simulink model "UdpHost"  (R2016b)
settings: Solver=FixedStepDiscrete  StartTime=0.0  StopTime=inf  FixedStep=CassieParameters.etherCatSampleTime  RelTol=1e-3  EnableMultiTasking=on
InitFcn:
  | udpInitFcn;
undefined symbols (not defined in the file or in its folder): inputBytes, outputBytes
libraries: ptplib x3, xpcutilitieslib x2
settings Model: xpc_rtwmakecfg_data=_xpciplib__xpcnblib__xpcetherlib__xpcether8255xlib__xpcetherGbElib_  SimulationMode=external  Creator=robot  LastModifiedBy=mikha
settings SolverCC: EnableConcurrentExecution=on  ConcurrentTasks=on
settings DataIOCC: SaveFormat=Array  SaveOutput=off  SignalLogging=off  DSMLogging=off  VisualizeSimOutput=off  SaveTime=off
settings OptimizationCC: DefaultParameterBehavior=Inlined  OptimizeBlockIOStorage=off  BufferReuse=off  GlobalBufferReuse=off  ExpressionFolding=off  LocalBlockOutputs=off  LifeSpan=inf  SimCompilerOptimization=on  AccelVerboseBuild=on
settings DebuggingCC: AllowSymbolicDim=off  SFUnexpectedBacktrackingDiag=warning  SFNoUnconditionalDefaultTransitionDiag=warning  SFExecutionAtInitializationDiag=none
settings HardwareCC: ProdBitPerPointer=32  ProdBitPerSizeT=32  ProdBitPerPtrDiffT=32  ProdLargestAtomicFloat=None  ProdWordSize=32  ProdLongLongMode=on  ProdHWDeviceType=Generic->32-bit x86 compatible
settings ModelReferenceCC: EnableParallelModelReferenceBuilds=on  ParallelModelReferenceMATLABWorkerInit=Copy Base Workspace  ModelReferenceNumInstancesAllowed=Zero  PropagateSignalLabelsOutOfModel=off
settings SFSimCC: SFSimEcho=off
settings RTWCC: SystemTargetFile=slrt.tlc  TLCOptions=-axPCMaxOverloads=1000000000 -axPCMaxOverloadLen=1000000000  TemplateMakefile=slrt_default_tmf  Description=Simulink Real-Time  RTWCompilerOptimization=on
settings CodeAppCC: GenerateComments=off  SimulinkBlockComments=off
settings SimulinkRealTimeCC: xPCTargetPCEnvName=NUC
settings ConfigComp: CovMetricSettings=dw  CovHtmlReporting=on  CovSaveCumulativeToWorkspaceVar=on  CovSaveSingleToWorkspaceVar=on  CovExternalEMLEnable=off

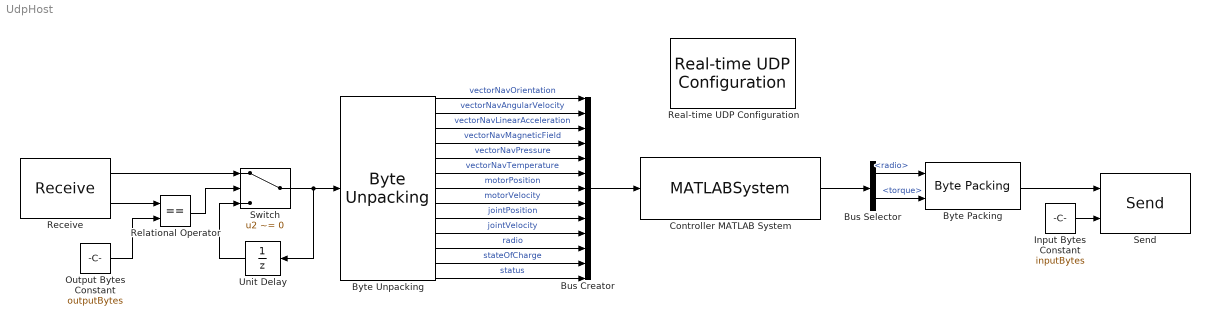
== system UdpHost ==
  Bus Creator : BusCreator  Inputs=13  OutDataTypeStr=Bus: cassieOutputsBus
  Bus Selector : BusSelector  OutputSignals=radio,torque
  "Byte Packing " : xpcutilitieslib/Byte Packing   MaskPackedDataType=uint8  MaskUnpackedDataTypes=inputTypes  MaskAlignment=1
  "Byte Unpacking " : xpcutilitieslib/Byte Unpacking   MaskUnpackedDataTypes=outputTypes  MaskUnpackedDataSizes=outputSizes  MaskAlignment=1
  Controller MATLAB System : MATLABSystem  System=NullController  SimulateUsing=Code generation
      mask Type: NullController
      mask Display:
      | disp('NullController');
      | port_label('input',1,'outputs');
      | port_label('output',1,'inputs');
  Input Bytes Constant : Constant  Value=inputBytes
  Output Bytes Constant : Constant  Value=outputBytes
  "Real-time UDP Configuration " : ptplib/PTP UDP/Real-time UDP  Configuration   ID=1  IpAddress=10.10.10.2  SubnetMask=255.255.255.0  Gateway=0.0.0.0  EthDrv=Intel Gigabit  PciBus=3  PciSlot=0  udpID=0  MulticastList=[]  Multicast={}
  "Receive " : ptplib/PTP UDP/Receive   ID=1  Receive1=0.0.0.0  Receive2=25000  Receive3=outputBytes  Receive4=-1  udpID=0
  Relational Operator : RelationalOperator  Operator===  OutDataTypeStr=boolean  RndMeth=Simplest
  "Send " : ptplib/PTP UDP/Send   ID=1  Send1=255.255.255.255  Send2=25001  Send3=-1  Send4=-1  udpID=0
  Switch : Switch  Criteria=u2 ~= 0
  Unit Delay : UnitDelay  SampleTime=-1
  wires:
  Controller MATLAB System/1 -> Bus Selector/1
  Bus Selector/1 -> "Byte Packing "/1  "<radio>"
  Bus Selector/2 -> "Byte Packing "/2  "<torque>"
  Relational Operator/1 -> Switch/2
  Switch/1 -> Unit Delay/1, "Byte Unpacking "/1
  Unit Delay/1 -> Switch/3
  "Receive "/2 -> Relational Operator/1
  "Receive "/1 -> Switch/1
  "Byte Packing "/1 -> "Send "/1
  Input Bytes Constant/1 -> "Send "/2
  Output Bytes Constant/1 -> Relational Operator/2
  Bus Creator/1 -> Controller MATLAB System/1
  "Byte Unpacking "/1 -> Bus Creator/1  "vectorNavOrientation"
  "Byte Unpacking "/2 -> Bus Creator/2  "vectorNavAngularVelocity"
  "Byte Unpacking "/3 -> Bus Creator/3  "vectorNavLinearAcceleration"
  "Byte Unpacking "/4 -> Bus Creator/4  "vectorNavMagneticField"
  "Byte Unpacking "/5 -> Bus Creator/5  "vectorNavPressure"
  "Byte Unpacking "/6 -> Bus Creator/6  "vectorNavTemperature"
  "Byte Unpacking "/7 -> Bus Creator/7  "motorPosition"
  "Byte Unpacking "/8 -> Bus Creator/8  "motorVelocity"
  "Byte Unpacking "/9 -> Bus Creator/9  "jointPosition"
  "Byte Unpacking "/10 -> Bus Creator/10  "jointVelocity"
  "Byte Unpacking "/11 -> Bus Creator/11  "radio"
  "Byte Unpacking "/12 -> Bus Creator/12  "stateOfCharge"
  "Byte Unpacking "/13 -> Bus Creator/13  "status"
